simulink model "PID_Controller_PS"  (R2020a)
settings: Solver=VariableStepAuto  StartTime=0.0  StopTime=120  RelTol=1e-3
model mask{Kd=1, Ki=60, Kp=1}
  mask prompts: Kd "Derivative Gain (Kd)"; Ki "Integral Gain (Ki)"; Kp "Proportional Gain (Kp)"
model workspace (MAT data in the model file):
  Kd = 1
  Ki = 60
  Kp = 1
settings Model: DataDictionary=Datadictionary_CruiseControl.sldd  ParameterArgumentNames=Kd,Ki,Kp  Creator=DELL  LastModifiedBy=DELL
settings DataIOCC: SaveOutput=off  SaveTime=off

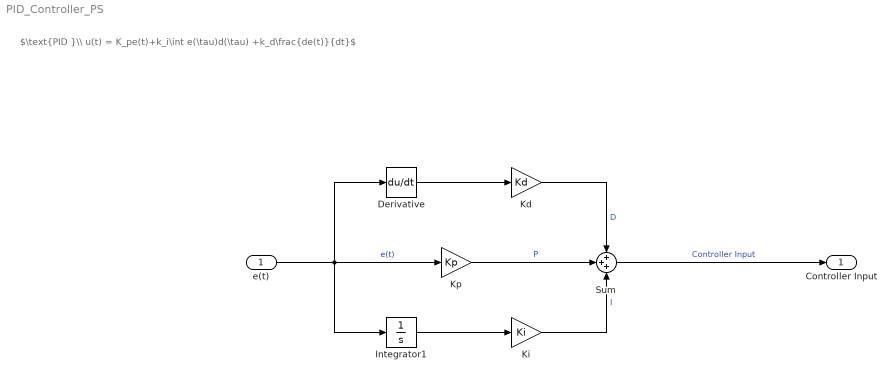
== system PID_Controller_PS ==
  note: $\text{PID }\\ u(t) = K_pe(t)+k_i\int e(\tau)d(\tau) +k_d\frac{de(t)}{dt}$
  e(t) : Inport  OutDataTypeStr=double  PortDimensions=1  SampleTime=0
  Derivative : Derivative
  Integrator1 : Integrator
  Kd : Gain  Gain=Kd
  Ki : Gain  Gain=Ki
  Kp : Gain  Gain=Kp
  Sum : Sum  Inputs=+++
  Controller Input : Outport  OutDataTypeStr=double  PortDimensions=1  SampleTime=0
  wires:
  Sum/1 -> Controller Input/1  "Controller Input"
  Kp/1 -> Sum/2  "P"
  Kd/1 -> Sum/1  "D"
  e(t)/1 -> Derivative/1, Kp/1, Integrator1/1  "e(t)"
  Ki/1 -> Sum/3  "I"
  Integrator1/1 -> Ki/1
  Derivative/1 -> Kd/1
